simulink model "sampleModel1514"  (R2023a)
settings: Solver=VariableStepAuto  StartTime=0.0  StopTime=10.0  RelTol=1e-3
libraries: hdlsllib x5, simulink x2
settings Model: Creator=user1  LastModifiedBy=user1

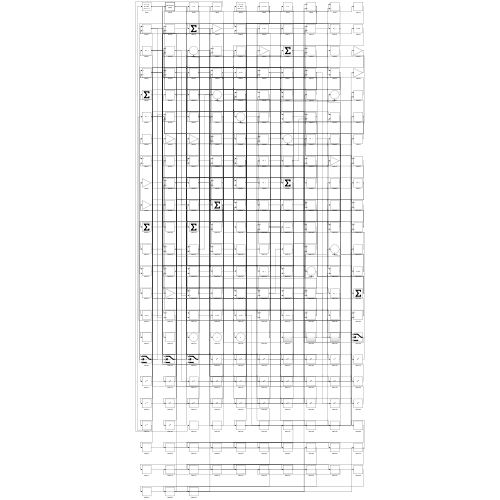
[thumbnail: Simulink's stored preview of the top-level diagram]
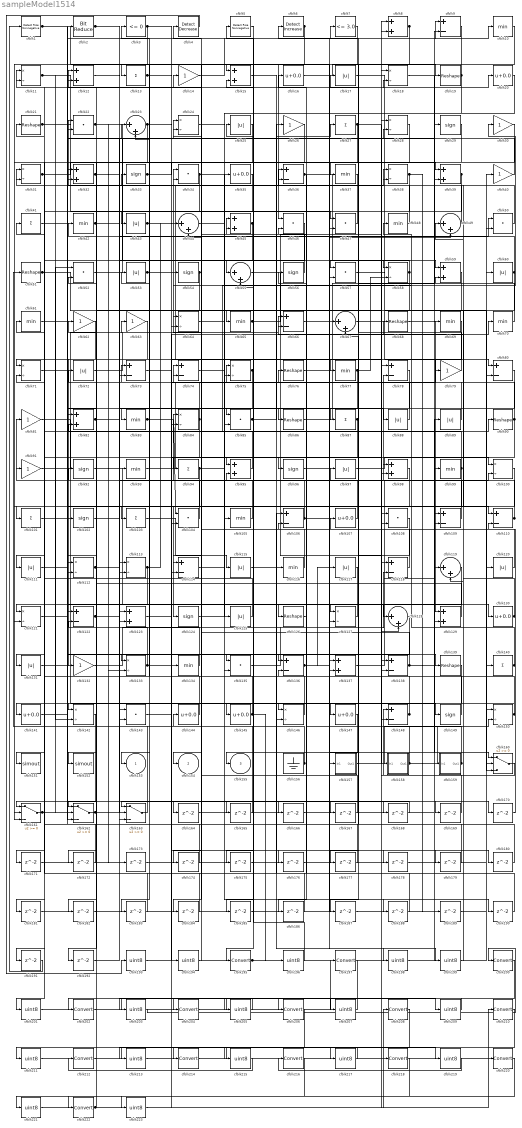
== system sampleModel1514 ==
  cfblk1 : hdlsllib/Logic and Bit Operations/Detect Rise Nonnegative  vinit=0  OutDataTypeStr=boolean
  cfblk{10,37,42,48,61,65,69..70,77,83,93,99,105,116,134} (15 alike) : MinMax
  cfblk{11,18,24,28,31,38,58,64,71,75,84,100,112..113,121,127,133,142,146,150} (20 alike) : Product  Inputs=*/  RndMeth=Zero  SaturateOnIntegerOverflow=on
  cfblk{13,27,41,87,94,101,103,140} (8 alike) : Sum  Inputs=+
  cfblk{29,33,54,56,92,96,102,124,149} (9 alike) : Signum
  cfblk{22,34,46..47,50,52,57,85,104,108,135,143} (12 alike) : DotProduct  OutDataTypeStr=Inherit: Inherit via internal rule
  cfblk{9,36,66,73..74,78,80,106,109..110,114,118,122,136,138,148} (16 alike) : Sum  Inputs=+-
  cfblk{16,20,35,107,130,141,144..145,147} (9 alike) : Bias  Bias=0.0  SaturateOnIntegerOverflow=off
  cfblk{17,25,43,53,60,72,88..89,97,111,115,117,120,125,131} (15 alike) : Abs  SaturateOnIntegerOverflow=off
  cfblk{23,44,49,55,67,119,128} (7 alike) : Sum  Inputs=|++
  cfblk{8,12,15,32,39,45,59,82,95,98,123,129,137} (13 alike) : Sum
  cfblk{19,21,51,68,76,86,90,126,139} (9 alike) : Reshape
  cfblk{14,26,30,40,62..63,79,81,91,132} (10 alike) : Gain
  cfblk151 : ToWorkspace  VariableName=simout  SaveFormat=Timeseries  SampleTime=-1
  cfblk152 : ToWorkspace  VariableName=simout  SaveFormat=Timeseries  SampleTime=-1
  cfblk156 : Ground
  cfblk157 : Subsystem
      settings: LibrarySourceBlock=|
      | hdlsllib/Ports &
      | Subsystems/Subsystem
  cfblk158 : Subsystem
      settings: LibrarySourceBlock=|
      | hdlsllib/Ports &
      | Subsystems/Subsystem
  cfblk159 : Subsystem
      settings: LibrarySourceBlock=|
      | hdlsllib/Ports &
      | Subsystems/Subsystem
  cfblk{160..163} (4 alike) : Switch  SaturateOnIntegerOverflow=off  InputSameDT=off
  cfblk{164..192} (29 alike) : Delay  SampleTime=1
  cfblk{193..194,196,198..199,201,203,205,207,209,211,213,215,217,219,221,223} (17 alike) : DataTypeConversion  OutDataTypeStr=uint8  SaturateOnIntegerOverflow=off  RndMeth=Floor
  cfblk{195,197,200,202,204,206,208,210,212,214,216,218,220,222} (14 alike) : DataTypeConversion  SaturateOnIntegerOverflow=off  RndMeth=Floor
  cfblk2 : hdlsllib/Logic and Bit Operations/Bit Reduce  mode=AND
  cfblk3 : hdlsllib/Logic and Bit Operations/Compare To Zero  relop=<=  OutDataTypeStr=boolean
  cfblk4 : simulink/Logic and Bit Operations/Detect Decrease  vinit=0.0  OutDataTypeStr=boolean
      settings: LibrarySourceBlock=|
      | hdlsllib/Logic and Bit
      | Operations/Detect
      | Decrease
  cfblk5 : hdlsllib/Logic and Bit Operations/Detect Rise Nonnegative  vinit=0  OutDataTypeStr=boolean
  cfblk6 : simulink/Logic and Bit Operations/Detect Increase  vinit=0.0  OutDataTypeStr=boolean
      settings: LibrarySourceBlock=|
      | hdlsllib/Logic and Bit
      | Operations/Detect
      | Increase
  cfblk7 : hdlsllib/Logic and Bit Operations/Compare To Constant  relop=<=  const=3.0  OutDataTypeStr=boolean
  cfblk153 : Outport  VectorParamsAs1DForOutWhenUnconnected=off
  cfblk154 : Outport  Port=2  VectorParamsAs1DForOutWhenUnconnected=off
  cfblk155 : Outport  Port=3  VectorParamsAs1DForOutWhenUnconnected=off
  wires:
  cfblk81/1 -> cfblk149/1
  cfblk127/1 -> cfblk121/1
  cfblk88/1 -> cfblk75/1
  cfblk115/1 -> cfblk116/1
  cfblk60/1 -> cfblk42/1, cfblk109/1, cfblk155/1
  cfblk163/1 -> cfblk51/1
  cfblk94/1 -> cfblk124/1, cfblk161/3, cfblk130/1
  cfblk56/1 -> cfblk11/1
  cfblk62/1 -> cfblk132/1
  cfblk67/1 -> cfblk129/1
  cfblk158/1(Out1) -> cfblk97/1, cfblk56/1
  cfblk160/1 -> cfblk148/1
  cfblk91/1 -> cfblk63/1
  cfblk95/1 -> cfblk30/1
  cfblk90/1 -> cfblk33/1, cfblk182/1, cfblk183/1
  cfblk58/1 -> cfblk57/1, cfblk64/2
  cfblk30/1 -> cfblk153/1
  cfblk97/1 -> cfblk100/1
  cfblk5/1 -> cfblk195/1
  cfblk156/1 -> cfblk144/1, cfblk52/2
  cfblk92/1 -> cfblk126/1
  cfblk87/1 -> cfblk142/1, cfblk192/1
  cfblk22/1 -> cfblk59/1, cfblk133/2
  cfblk145/1 -> cfblk74/1, cfblk44/2, cfblk196/1
  cfblk7/1 -> cfblk95/1
  cfblk113/1 -> cfblk162/1, cfblk44/1, cfblk23/2
  cfblk28/1 -> cfblk122/1
  cfblk79/1 -> cfblk6/1
  cfblk19/1 -> cfblk15/1, cfblk145/1
  cfblk26/1 -> cfblk82/1
  cfblk86/1 -> cfblk29/1
  cfblk146/1 -> cfblk12/1
  cfblk104/1 -> cfblk81/1
  cfblk157/1(Out1) -> cfblk150/2
  cfblk6/1 -> cfblk83/1, cfblk161/2
  cfblk110/1 -> cfblk78/2, cfblk53/1
  cfblk16/1 -> cfblk19/1
  cfblk141/1 -> cfblk20/1
  cfblk93/1 -> cfblk69/1
  cfblk11/1 -> cfblk105/1, cfblk142/2, cfblk138/2
  cfblk140/1 -> cfblk59/2, cfblk54/1, cfblk48/1
  cfblk24/1 -> cfblk125/1
  cfblk116/1 -> cfblk25/1
  cfblk120/1 -> cfblk45/1
  cfblk149/1 -> cfblk91/1
  cfblk138/1 -> cfblk99/1, cfblk64/1, cfblk189/1
  cfblk132/1 -> cfblk100/2
  cfblk68/1 -> cfblk80/1
  cfblk48/1 -> cfblk22/1
  cfblk55/1 -> cfblk158/1(In1)
  cfblk82/1 -> cfblk110/1, cfblk148/2
  cfblk41/1 -> cfblk86/1
  cfblk46/1 -> cfblk75/2
  cfblk36/1 -> cfblk118/1, cfblk88/1, cfblk186/1
  cfblk69/1 -> cfblk102/1
  cfblk103/1 -> cfblk115/1
  cfblk1/1 -> cfblk67/1, cfblk139/1
  cfblk133/1 -> cfblk62/1, cfblk178/1
  cfblk76/1 -> cfblk157/1(In1)
  cfblk9/1 -> cfblk65/1
  cfblk10/1 -> cfblk46/1
  cfblk31/1 -> cfblk37/1, cfblk36/2, cfblk108/2, cfblk127/2
  cfblk8/1 -> cfblk147/1, cfblk114/1
  cfblk54/1 -> cfblk112/1, cfblk94/1
  cfblk161/1 -> cfblk9/1, cfblk52/1
  cfblk143/1 -> cfblk79/1
  cfblk27/1 -> cfblk151/1, cfblk109/2
  cfblk32/1 -> cfblk93/1, cfblk164/1
  cfblk134/1 -> cfblk23/1
  cfblk51/1 -> cfblk113/2, cfblk134/1, cfblk128/2
  cfblk70/1 -> cfblk17/1
  cfblk85/1 -> cfblk27/1, cfblk190/1
  cfblk118/1 -> cfblk24/1
  cfblk130/1 -> cfblk31/1, cfblk66/1
  cfblk135/1 -> cfblk118/2
  cfblk112/1 -> cfblk66/2, cfblk172/1, cfblk173/1
  cfblk59/1 -> cfblk146/1
  cfblk23/1 -> cfblk121/2, cfblk85/1, cfblk39/2
  cfblk109/1 -> cfblk45/2
  cfblk111/1 -> cfblk24/2
  cfblk101/1 -> cfblk90/1
  cfblk96/1 -> cfblk160/1
  cfblk14/1 -> cfblk7/1
  cfblk66/1 -> cfblk10/1
  cfblk125/1 -> cfblk61/1
  cfblk83/1 -> cfblk104/1, cfblk176/1
  cfblk148/1 -> cfblk46/2, cfblk55/2
  cfblk17/1 -> cfblk160/2
  cfblk52/1 -> cfblk9/2
  cfblk78/1 -> cfblk123/2
  cfblk128/1 -> cfblk162/3
  cfblk139/1 -> cfblk154/1
  cfblk126/1 -> cfblk36/1
  cfblk137/1 -> cfblk89/1
  cfblk150/1 -> cfblk21/1, cfblk141/1
  cfblk71/1 -> cfblk2/1
  cfblk21/1 -> cfblk143/1, cfblk84/2, cfblk18/2, cfblk85/2
  cfblk18/1 -> cfblk160/3
  cfblk72/1 -> cfblk34/1
  cfblk34/1 -> cfblk103/1, cfblk57/2
  cfblk159/1(Out1) -> cfblk107/1, cfblk106/2
  cfblk50/1 -> cfblk16/1
  cfblk33/1 -> cfblk39/1, cfblk98/2
  cfblk75/1 -> cfblk74/2, cfblk143/2, cfblk133/1
  cfblk84/1 -> cfblk12/2, cfblk131/1
  cfblk105/1 -> cfblk95/2
  cfblk38/1 -> cfblk127/1, cfblk114/2, cfblk159/1(In1)
  cfblk123/1 -> cfblk68/1
  cfblk65/1 -> cfblk135/1, cfblk8/1
  cfblk63/1 -> cfblk161/1
  cfblk3/1 -> cfblk13/1, cfblk137/2
  cfblk122/1 -> cfblk136/1, cfblk92/1, cfblk152/1
  cfblk106/1 -> cfblk41/1, cfblk49/2, cfblk170/1, cfblk179/1
  cfblk61/1 -> cfblk14/1
  cfblk39/1 -> cfblk184/1, cfblk185/1
  cfblk57/1 -> cfblk140/1
  cfblk162/1 -> cfblk98/1, cfblk28/2
  cfblk99/1 -> cfblk31/2, cfblk111/1
  cfblk49/1 -> cfblk3/1
  cfblk2/1 -> cfblk47/1, cfblk55/1
  cfblk74/1 -> cfblk35/1
  cfblk144/1 -> cfblk73/1
  cfblk43/1 -> cfblk26/1, cfblk77/1
  cfblk45/1 -> cfblk112/2, cfblk171/1
  cfblk89/1 -> cfblk76/1
  cfblk129/1 -> cfblk32/2
  cfblk47/1 -> cfblk43/1
  cfblk53/1 -> cfblk38/1, cfblk108/1
  cfblk40/1 -> cfblk22/2
  cfblk102/1 -> cfblk50/1
  cfblk25/1 -> cfblk71/1
  cfblk124/1 -> cfblk70/1
  cfblk77/1 -> cfblk96/1, cfblk58/2
  cfblk13/1 -> cfblk146/2, cfblk180/1
  cfblk80/1 -> cfblk163/2
  cfblk136/1 -> cfblk38/2, cfblk117/1
  cfblk20/1 -> cfblk135/2
  cfblk44/1 -> cfblk87/1
  cfblk42/1 -> cfblk128/1, cfblk58/1
  cfblk107/1 -> cfblk84/1
  cfblk29/1 -> cfblk73/2
  cfblk37/1 -> cfblk101/1
  cfblk164/1 -> cfblk129/2
  cfblk98/1 -> cfblk165/1
  cfblk165/1 -> cfblk113/1
  cfblk121/1 -> cfblk166/1
  cfblk114/1 -> cfblk167/1
  cfblk167/1 -> cfblk34/2
  cfblk12/1 -> cfblk168/1
  cfblk168/1 -> cfblk163/1
  cfblk131/1 -> cfblk169/1
  cfblk169/1 -> cfblk78/1
  cfblk170/1 -> cfblk110/2
  cfblk171/1 -> cfblk80/2
  cfblk172/1 -> cfblk162/2
  cfblk173/1 -> cfblk47/2
  cfblk35/1 -> cfblk174/1
  cfblk174/1 -> cfblk32/1
  cfblk147/1 -> cfblk175/1
  cfblk175/1 -> cfblk15/2
  cfblk176/1 -> cfblk28/1
  cfblk100/1 -> cfblk177/1
  cfblk177/1 -> cfblk122/2
  cfblk178/1 -> cfblk50/2
  cfblk179/1 -> cfblk67/2
  cfblk180/1 -> cfblk71/2
  cfblk142/1 -> cfblk181/1
  cfblk181/1 -> cfblk137/1
  cfblk182/1 -> cfblk18/1
  cfblk183/1 -> cfblk11/2
  cfblk184/1 -> cfblk82/2
  cfblk185/1 -> cfblk138/1
  cfblk186/1 -> cfblk106/1
  cfblk108/1 -> cfblk187/1
  cfblk187/1 -> cfblk150/1
  cfblk64/1 -> cfblk188/1
  cfblk188/1 -> cfblk123/1
  cfblk189/1 -> cfblk49/1
  cfblk190/1 -> cfblk136/2
  cfblk117/1 -> cfblk191/1
  cfblk191/1 -> cfblk1/1
  cfblk192/1 -> cfblk163/3
  cfblk4/1 -> cfblk193/1
  cfblk193/1 -> cfblk120/1
  cfblk73/1 -> cfblk194/1
  cfblk194/1 -> cfblk4/1
  cfblk195/1 -> cfblk60/1, cfblk40/1
  cfblk196/1 -> cfblk5/1
  cfblk15/1 -> cfblk198/1
  cfblk198/1 -> cfblk119/1
  cfblk166/1 -> cfblk199/1
  cfblk199/1 -> cfblk119/2
  cfblk119/1 -> cfblk201/1
  cfblk201/1 -> cfblk197/1
  cfblk197/1 -> cfblk203/1
  cfblk203/1 -> cfblk200/1
  cfblk200/1 -> cfblk205/1
  cfblk205/1 -> cfblk202/1
  cfblk202/1 -> cfblk207/1
  cfblk207/1 -> cfblk204/1
  cfblk204/1 -> cfblk209/1
  cfblk209/1 -> cfblk206/1
  cfblk206/1 -> cfblk211/1
  cfblk211/1 -> cfblk208/1
  cfblk208/1 -> cfblk213/1
  cfblk213/1 -> cfblk210/1
  cfblk210/1 -> cfblk215/1
  cfblk215/1 -> cfblk212/1
  cfblk212/1 -> cfblk217/1
  cfblk217/1 -> cfblk214/1
  cfblk214/1 -> cfblk219/1
  cfblk219/1 -> cfblk216/1
  cfblk220/1 -> cfblk222/1
  cfblk216/1 -> cfblk221/1
  cfblk221/1 -> cfblk218/1
  cfblk222/1 -> cfblk8/2, cfblk104/2, cfblk72/1
  cfblk218/1 -> cfblk223/1
  cfblk223/1 -> cfblk220/1

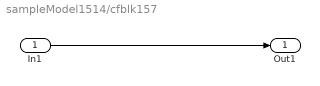
== system sampleModel1514/cfblk157 ==
  In1 : Inport
  Out1 : Outport
  wires:
  In1/1 -> Out1/1

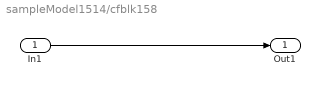
== system sampleModel1514/cfblk158 ==
  In1 : Inport
  Out1 : Outport
  wires:
  In1/1 -> Out1/1

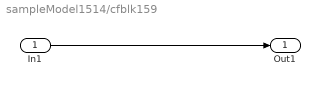
== system sampleModel1514/cfblk159 ==
  In1 : Inport
  Out1 : Outport
  wires:
  In1/1 -> Out1/1
